simulink model "MotorControl_5"  (Simulink 8.1)
settings: Solver=FixedStepDiscrete  StartTime=0.0  StopTime=50  FixedStep=0.5  RelTol=1e-3
PostLoadFcn:
  | MotorControl_5_data
undefined symbols (not defined in the file or in its folder): A14, B, B13, D, L3, R10
libraries: BAMLIB564xL x4, rappid_564xl_ec_toolbox x1
settings Model: Creator=evarshavskaya  LastModifiedBy=evarshavskaya
settings DataIOCC: ExternalInput=off  InitialState=off  SaveOutput=off  SignalLogging=off  SaveTime=off
settings OptimizationCC: InlineParams=on  OptimizeModelRefInitCode=on  LifeSpan=1
settings DebuggingCC: InheritedTsInSrcMsg=none  SingleTaskRateTransMsg=error  ParameterPrecisionLossMsg=none  UnconnectedInputMsg=error  UnconnectedOutputMsg=error  UnconnectedLineMsg=error  UnknownTsInhSupMsg=error
settings HardwareCC: ProdLargestAtomicInteger=Long  ProdLargestAtomicFloat=Double  ProdIntDivRoundTo=Zero  ProdEndianess=BigEndian  ProdHWDeviceType=Freescale->32-bit PowerPC
settings RTWCC: SystemTargetFile=rappid564xl.tlc  MakeCommand=rappid_564xl_make_rtw  TemplateMakefile=rappid_564xl_default_tmf  PostCodeGenCommand=rappid_analyzegencode(buildInfo)  Description=RAppID Toolbox MPC564xL Code Generation Target (rappid)  RetainRTWFile=on  ProcessScript=rappid564xl_make_rtw_hook
settings CodeAppCC: IgnoreCustomStorageClasses=off  CustomSymbolStrType=$N$R$M  InternalIdentifier=Classic
settings STFCustomTargetCC: CodeReplacementLibrary=ANSI_C  ModelReferenceCompliant=off  CombineOutputUpdateFcns=on  SuppressErrorStatus=on  ERTCustomFileBanners=on  SupportContinuousTime=off  SupportNonInlinedSFcns=off  MATLABClassNameForMDSCustomization=Simulink.SoftwareTarget.ERTCustomization  GRTInterface=off  SystemTargetFile=rappid564xl.tlc
settings ERTTargetCC: CodeReplacementLibrary=ANSI_C  MultiwordLength=2048  ModelReferenceCompliant=off  ParMdlRefBuildCompliant=off  CompOptLevelCompliant=off  ConcurrentExecutionCompliant=off  SuppressErrorStatus=on  ERTFirstTimeCompliant=off  ModelStepFunctionPrototypeControlCompliant=off  CPPClassGenCompliant=off  ExtModeMexFile=noextcomm  InlinedParameterPlacement=NonHierarchical  ERTCustomFileTemplate=example_file_process.tlc  ConvertIfToSwitch=off  SuppressUnreachableDefaultCases=off

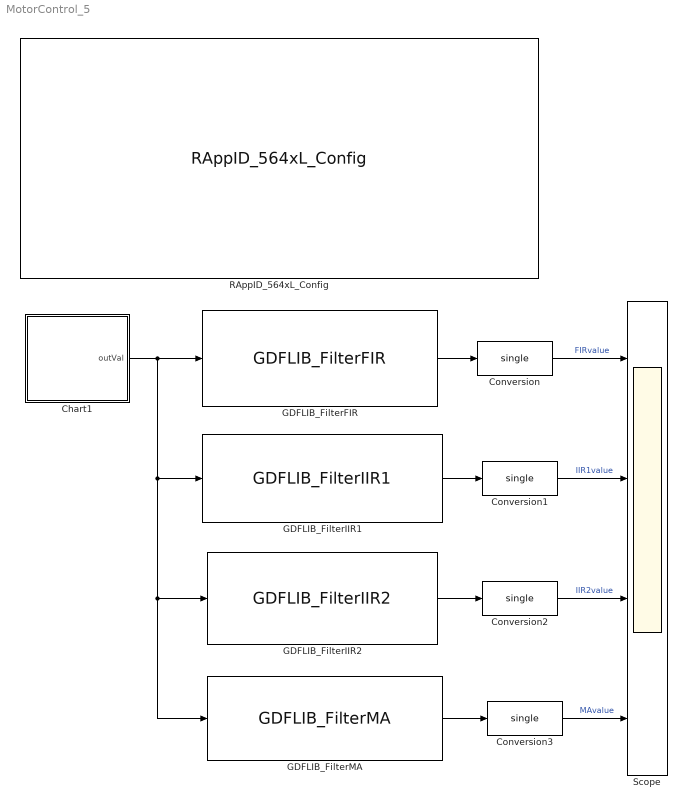
== system MotorControl_5 ==
  Chart1 : Stateflow chart  TreatAsAtomicUnit=on
  Conversion{,1..3} (4 alike) : DataTypeConversion  OutDataTypeStr=single
  GDFLIB_FilterFIR : BAMLIB564xL/General Digital Filters/GDFLIB_FilterFIR  u32Order=Order  ps32CoefBuf=CoefBuf
  GDFLIB_FilterIIR1 : BAMLIB564xL/General Digital Filters/GDFLIB_FilterIIR1  s32B0=s32B0  s32B1=s32B1  s32A1=s32A1
  GDFLIB_FilterIIR2 : BAMLIB564xL/General Digital Filters/GDFLIB_FilterIIR2  s32B0=s32B0_2  s32B1=s32B1_2  s32B2=s32B2_2  s32A1=s32A1_2  s32A2=s32A2_2
  GDFLIB_FilterMA : BAMLIB564xL/General Digital Filters/GDFLIB_FilterMA  u16NSamples=u16NSamples
  RAppID_564xL_Config : rappid_564xl_ec_toolbox/MPC564xL/RAppID_564xL_Config  SystemClock=120  XTAL=40  MC_clock_60=12  MC_clock_80=16  MC_clock_120=10  SWG_clock_60=20  SWG_clock_80=13.334  SWG_clock_120=20  Compiler=CodeWarrior  MemTarget=RAM  Part=MPC5643L  Package=144 LQFP  global_int_priority=10  base_tick_priority=14  sys_task_supress=off  exception_handlers=off  stored_mdl_name=MotorControl_5  freemaster_interface=Oops  freemaster_rx_pin="LINFlex_0 Rx Pin 116 : \"PB[3]\""  freemaster_tx_pin="LINFlex_0 Tx Pin 114 : \"PB[2]\""  freemaster_interface_1=Serial 0  freemaster_enable=on  freemaster_rate=57600  freemaster_tx0_pin=18 : B[2] : 114 : A14  freemaster_rx0_pin=19 : B[3] : 116 : B13  freemaster_tx1_pin=57 : D[9] : 26 : L3  freemaster_rx1_pin=29 : B[13] : 60 : R10  freemaster_can_channel=1CH  freemater_can_speed=500K  freemaster_can_msgig=0x7AA  ccp_interface=None  ccp_enable=off  ccp_can_channel=CH1 (MB 0 - 1)  ccp_can_speed=500K  ccp_can_cro_id=256  ccp_can_dto_id=257  ccp_dev_id=RappID  ccp_dev_addr=0  ccp_odt=3  ccp_daq=3  pil_enable=off  pil_bam=on  comport=1  pil_rate=57600  bam_password_def=on  bam_password=0xFEEDFACECAFEBEEF  bam_sa_cs=off  bam_start_address=0x0  bam_code_size=0x7000  cons_dspi=on  cons_can=on  cons_adc=on  cons_pwm=on  cons_ctu=on  cons_swg=on  cons_eTimer=on  cons_fm=on
  Scope : Scope  NumInputPorts=4
      settings: TimeRange=50  YMin=-5~-1~-1.5~-0.5  YMax=5~1~1.5~0.5
  wires:
  Chart1/1(outVal) -> GDFLIB_FilterFIR/1, GDFLIB_FilterIIR1/1, GDFLIB_FilterIIR2/1, GDFLIB_FilterMA/1
  GDFLIB_FilterFIR/1 -> Conversion/1
  Conversion/1 -> Scope/1  "FIRvalue"
  GDFLIB_FilterIIR1/1 -> Conversion1/1
  Conversion1/1 -> Scope/2  "IIR1value"
  GDFLIB_FilterIIR2/1 -> Conversion2/1
  Conversion2/1 -> Scope/3  "IIR2value"
  GDFLIB_FilterMA/1 -> Conversion3/1
  Conversion3/1 -> Scope/4  "MAvalue"

== stateflow chart Chart1 ==
  settings: executeAtInitialization=1
  state A
    du:
    outVal =1;
    cntr=cntr+1;
  state A1
    du:
    outVal =-1;
    cntr=cntr-1;
  (default) -> A : {cntr=0;}
  A1 -> A : [cntr < 2]
  A -> A1 : [cntr > 10]
  data: cntr local uint32 [0..12] =0; outVal output single [-1..1]
